simulink model "yaw_control"  (R2021a)
settings: Solver=VariableStepAuto  StartTime=0  StopTime=10  RelTol=R_tol
values from neighbouring files (symbols this model uses):
  Iry = 0.07    [auto_sim.m]
  Iz = 0.9    [auto_sim.m]
  K1 = (16/T_s(i)^2)*(pi^2/log(OS(i)/100)^2+1)    [auto_sim.m]
  K2 = 8/T_s(i)    [auto_sim.m]
  Kmoi = (Ix-Iy)/Ix*Iy*Iz    (= 0.2625)    [auto_sim.m]
  theta_dot = 9    [auto_sim.m]
settings Model: OrderedModelArguments=off  Creator=ezeor  LastModifiedBy=ezeor
settings DataIOCC: ExternalInput=[time_step, wind, wind_dot, wind_ddot]  LoadExternalInput=on

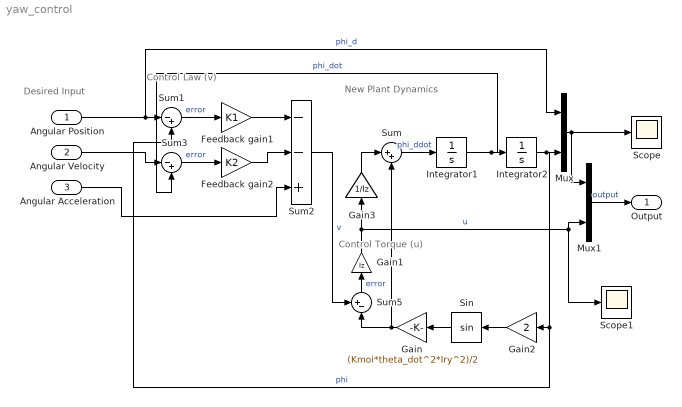
== system yaw_control ==
  note: New Plant Dynamics
  note: Control Torque (u)
  note: Desired Input
  note: Control Law (v)
  Angular Position : Inport
  Angular Velocity : Inport  Port=2
  Angular Acceleration : Inport  Port=3
  Feedback gain1 : Gain  Gain=K1
  Feedback gain2 : Gain  Gain=K2
  Gain : Gain  Gain=(Kmoi*theta_dot^2*Iry^2)/2
  Gain1 : Gain  Gain=Iz
  Gain2 : Gain  Gain=2
  Gain3 : Gain  Gain=1/Iz
  Integrator1 : Integrator
  Integrator2 : Integrator
  Mux : Mux  Inputs=2
  Mux1 : Mux  Inputs=2
  Scope : Scope
  Scope1 : Scope
  Sin : Trigonometry
  Sum : Sum  Inputs=|++
  Sum1 : Sum  Inputs=|-+
  Sum2 : Sum  Inputs=--+
  Sum3 : Sum  Inputs=|-+
  Sum5 : Sum  Inputs=+-|
  Output : Outport
  wires:
  Integrator1/1 -> Sum3/2, Integrator2/1  "phi_dot"
  Integrator2/1 -> Gain2/1, Sum1/2, Mux/2  "phi"
  Mux/1 -> Mux1/1, Scope/1
  Sum2/1 -> Sum5/1  "v"
  Feedback gain1/1 -> Sum2/1
  Angular Position/1 -> Sum1/1, Mux/1  "phi_d"
  Sum1/1 -> Feedback gain1/1  "error"
  Angular Velocity/1 -> Sum3/1
  Sum3/1 -> Feedback gain2/1  "error"
  Feedback gain2/1 -> Sum2/2
  Angular Acceleration/1 -> Sum2/3
  Sin/1 -> Gain/1
  Gain2/1 -> Sin/1
  Gain/1 -> Sum/2, Sum5/2
  Sum5/1 -> Gain1/1  "error"
  Gain1/1 -> Gain3/1, Scope1/1, Mux1/2  "u"
  Sum/1 -> Integrator1/1  "phi_ddot"
  Gain3/1 -> Sum/1
  Mux1/1 -> Output/1  "output"
